simulink model "SimTF"  (R2024b)
settings: Solver=VariableStepAuto  StartTime=0.0  StopTime=5  RelTol=1e-3
undefined symbols (not defined in the file or in its folder): den_tf, num_tf
settings Model: Creator=ematric  LastModifiedBy=ematric

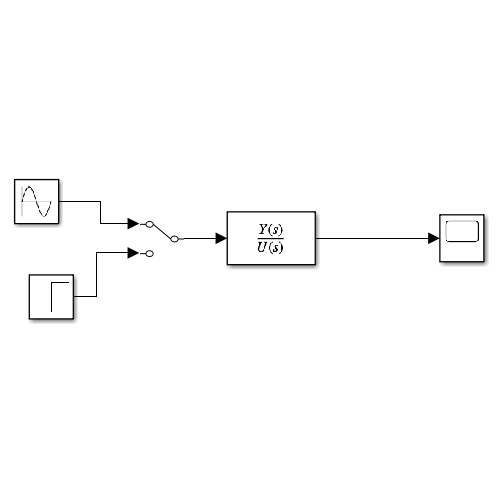
[thumbnail: Simulink's stored preview of the top-level diagram]
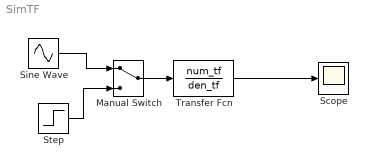
== system SimTF ==
  Manual Switch : ManualSwitch
  Scope : Scope
  Sine Wave : Sin  Amplitude=5  Frequency=252  SampleTime=0
  Step : Step  SampleTime=0
  Transfer Fcn : TransferFcn  Numerator=num_tf  Denominator=den_tf
  wires:
  Transfer Fcn/1 -> Scope/1
  Step/1 -> Manual Switch/2
  Manual Switch/1 -> Transfer Fcn/1
  Sine Wave/1 -> Manual Switch/1
